simulink model "main"  (R2017a)
settings: Solver=VariableStepAuto  StartTime=0.0  StopTime=0.26  FixedStep=2e-4  RelTol=1e-3
values from neighbouring files (symbols this model uses):
  accFir = c*[1 -2 1]    [initiateSimulation.m]
  F2 = denGpDis/sum(numGpDis)    [initiateSimulation.m]
  jerkFir = c*[1 -3 3 -1]    [initiateSimulation.m]
  snapFir = c*[1 -4 6 -4 1]    [initiateSimulation.m]
  totalMass = 25    [initiateSimulation.m]
  Ts = 1/fs    (= 0.0002)    [initiateSimulation.m]
  TsN = 1e-5    (= 1e-05)    [initiateSimulation.m]
undefined symbols (not defined in the file or in its folder): denGcDis, denGp, denIIR, numGcDis, numGp, numIIR
libraries: model_controller x2, simulink x1
settings Model: Creator=Dai Luyao  LastModifiedBy=Dai Luyao

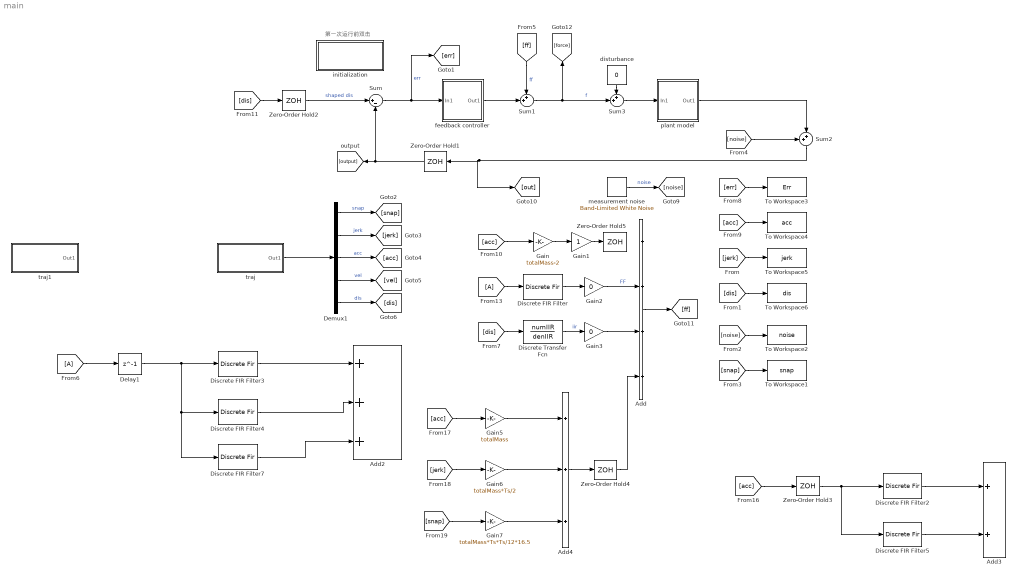
== system main ==
  note: 第一次运行前双击
  Add : Sum  Inputs=++++
  Add2 : Sum  Inputs=+++
  Add3 : Sum
  Add4 : Sum  Inputs=+++
  Delay1 : Delay  DelayLength=1  SampleTime=Ts
  Demux1 : Demux  Outputs=5
  Discrete Transfer Fcn : DiscreteTransferFcn  Numerator=numIIR  Denominator=denIIR  SampleTime=Ts
  Discrete FIR Filter : DiscreteFir  Coefficients=F2  SampleTime=Ts
  Discrete FIR Filter2 : DiscreteFir  Coefficients=totalMass  SampleTime=Ts
  Discrete FIR Filter3 : DiscreteFir  Coefficients=accFir  SampleTime=Ts
  Discrete FIR Filter4 : DiscreteFir  Coefficients=jerkFir*2.5  SampleTime=Ts
  Discrete FIR Filter5 : DiscreteFir  Coefficients=[1 -1]*totalMass/2  SampleTime=Ts
  Discrete FIR Filter7 : DiscreteFir  Coefficients=snapFir*24/4  SampleTime=Ts
  Gain : Gain  Gain=totalMass-2
  Gain1 : Gain
  Gain2 : Gain  Gain=0
  Gain3 : Gain  Gain=0
  Gain5 : Gain  Gain=totalMass
  Gain6 : Gain  Gain=totalMass*Ts/2
  Gain7 : Gain  Gain=totalMass*Ts*Ts/12*16.5
  Sum : Sum  Inputs=|+-
  Sum1 : Sum  Inputs=++|
  Sum2 : Sum  Inputs=++|
  Sum3 : Sum  Inputs=++|
  To Workspace1 : ToWorkspace  VariableName=snap  SaveFormat=Structure With Time  SampleTime=-1
  To Workspace2 : ToWorkspace  VariableName=noise  SaveFormat=Structure With Time  SampleTime=-1
  To Workspace3 : ToWorkspace  VariableName=Err  SaveFormat=Structure With Time  SampleTime=-1
  To Workspace4 : ToWorkspace  VariableName=acc  SaveFormat=Structure With Time  SampleTime=-1
  To Workspace5 : ToWorkspace  VariableName=jerk  SaveFormat=Structure With Time  SampleTime=-1
  To Workspace6 : ToWorkspace  VariableName=dis  SaveFormat=Structure With Time  SampleTime=-1
  Zero-Order Hold{1..5} (5 alike) : ZeroOrderHold  SampleTime=Ts
  disturbance : Constant  Value=0
  feedback controller : Subsystem
  initialization : Subsystem
      settings: OpenFcn=initiateSimulation;  MoveFcn=edit initiateSimulation;
  measurement noise : simulink/Sources/Band-Limited White Noise  Cov=noisePower  Ts=TsN  seed=[23341]
  plant model : Subsystem
  traj : Subsystem  BlockChoice=4th order traj
      link override 3rd order traj: j=800  v=0.25  x=0.06  a=10
      link override 4th order traj: a=10  v=0.25  j=800  d=64000
      settings: AttributesFormatString=%<BlockChoice>  TemplateBlock=model_controller/Profile Generators/traj  MemberBlocks=2nd order traj,3rd order traj,4th order traj,step,zero
  traj1 : Subsystem  BlockChoice=4th order traj
      link override 3rd order traj: j=800  v=0.25  x=0.06  a=10
      link override 4th order traj: a=20  v=0.5  x=0.05  j=2000  d=1.5e6
      settings: AttributesFormatString=%<BlockChoice>  TemplateBlock=model_controller/Profile Generators/traj  MemberBlocks=2nd order traj,3rd order traj,4th order traj,step,zero
  wires:
  Sum/1 -> feedback controller/1(In1), [err]  "err"
  Sum1/1 -> Sum3/2, [force]  "f"
  measurement noise/1 -> [noise]  "noise"
  Demux1/1 -> [snap]  "snap"
  Demux1/2 -> [jerk]  "jerk"
  Demux1/3 -> [acc]  "acc"
  Demux1/4 -> [vel]  "vel"
  Demux1/5 -> [dis]  "dis"
  [acc] -> To Workspace4/1
  [acc] -> Gain/1
  [jerk] -> To Workspace5/1
  [dis] -> To Workspace6/1
  [err] -> To Workspace3/1
  [noise] -> To Workspace2/1
  disturbance/1 -> Sum3/1
  Sum3/1 -> plant model/1(In1)
  plant model/1(Out1) -> Sum2/2
  Discrete FIR Filter/1 -> Gain2/1
  Add/1 -> [ff]
  Sum2/1 -> Zero-Order Hold1/1, [out]
  feedback controller/1(Out1) -> Sum1/2
  Gain2/1 -> Add/2  "FF"
  Discrete Transfer Fcn/1 -> Gain3/1  "iir"
  Gain3/1 -> Add/3
  [dis] -> Discrete Transfer Fcn/1
  Zero-Order Hold2/1 -> Sum/1  "shaped dis"
  Zero-Order Hold1/1 -> Sum/2, [output]
  [dis] -> Zero-Order Hold2/1
  [A] -> Discrete FIR Filter/1
  Gain/1 -> Gain1/1
  [noise] -> Sum2/1
  Discrete FIR Filter3/1 -> Add2/1
  Zero-Order Hold3/1 -> Discrete FIR Filter5/1, Discrete FIR Filter2/1
  Discrete FIR Filter2/1 -> Add3/1
  [acc] -> Zero-Order Hold3/1
  Discrete FIR Filter5/1 -> Add3/2
  Gain1/1 -> Zero-Order Hold5/1
  Discrete FIR Filter4/1 -> Add2/2
  [A] -> Delay1/1
  Delay1/1 -> Discrete FIR Filter7/1, Discrete FIR Filter4/1, Discrete FIR Filter3/1
  Discrete FIR Filter7/1 -> Add2/3
  Gain5/1 -> Add4/1
  [acc] -> Gain5/1
  [jerk] -> Gain6/1
  [snap] -> Gain7/1
  Gain7/1 -> Add4/3
  Add4/1 -> Zero-Order Hold4/1
  Gain6/1 -> Add4/2
  traj/1(Out1) -> Demux1/1
  [ff] -> Sum1/1  "ff"
  Zero-Order Hold4/1 -> Add/4
  [snap] -> To Workspace1/1

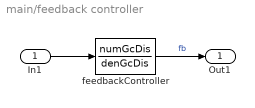
== system main/feedback controller ==
  In1 : Inport
  feedbackController : DiscreteTransferFcn  Numerator=numGcDis  Denominator=denGcDis  SampleTime=Ts
  Out1 : Outport
  wires:
  feedbackController/1 -> Out1/1  "fb"
  In1/1 -> feedbackController/1

== system main/initialization ==

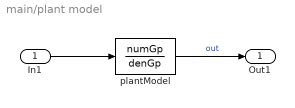
== system main/plant model ==
  In1 : Inport
  plantModel : TransferFcn  Numerator=numGp  Denominator=denGp
  Out1 : Outport
  wires:
  In1/1 -> plantModel/1
  plantModel/1 -> Out1/1  "out"

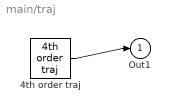
== system main/traj ==
  4th order traj : model_controller/Profile Generators/4th order traj  t0=0  x=0.05  v=0.25  a=10  j=800  d=64000  Ts=0
  Out1 : Outport
  wires:
  4th order traj/1 -> Out1/1

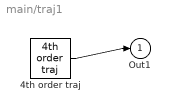
== system main/traj1 ==
  4th order traj : model_controller/Profile Generators/4th order traj  t0=0  x=0.05  v=0.5  a=20  j=2000  d=1.5e6  Ts=0
  Out1 : Outport
  wires:
  4th order traj/1 -> Out1/1
